simulink model "Line_Follower"  (R2024b)
settings: Solver=VariableStepAuto  StartTime=0.0  StopTime=360  RelTol=1e-3
settings Model: Creator=varun  LastModifiedBy=varun

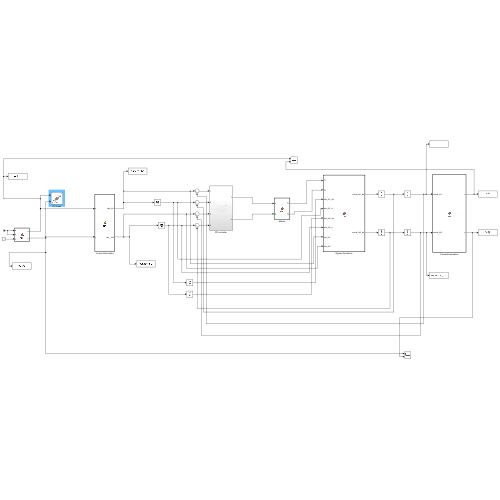
[thumbnail: Simulink's stored preview of the top-level diagram]
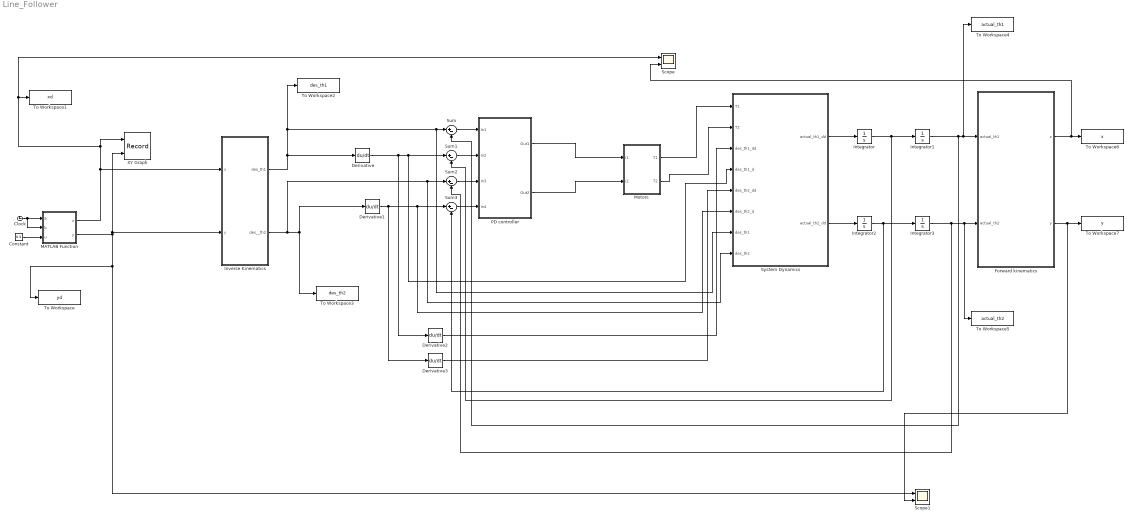
== system Line_Follower ==
  Clock : Clock
      settings: Decimation=360
  Constant : Constant  Value=0.3
  Derivative{,1..3} (4 alike) : Derivative
  Forward kinematics : MATLAB Function  TreatAsAtomicUnit=on
  Integrator{,1..3} (4 alike) : Integrator
  Inverse Kinematics : MATLAB Function  TreatAsAtomicUnit=on
  MATLAB Function : MATLAB Function  TreatAsAtomicUnit=on
  Motors : MATLAB Function  TreatAsAtomicUnit=on
  PD controller : Subsystem
  Scope : Scope  NumInputPorts=2
  Scope1 : Scope  NumInputPorts=2
  Sum{,1..3} (4 alike) : Sum  Inputs=|+-
  System Dynamics : MATLAB Function  TreatAsAtomicUnit=on
  To Workspace : ToWorkspace  VariableName=yd  SampleTime=-1
  To Workspace1 : ToWorkspace  VariableName=xd  SampleTime=-1
  To Workspace2 : ToWorkspace  VariableName=des_th1  SampleTime=-1
  To Workspace3 : ToWorkspace  VariableName=des_th2  SampleTime=-1
  To Workspace4 : ToWorkspace  VariableName=actual_th1  SampleTime=-1
  To Workspace5 : ToWorkspace  VariableName=actual_th2  SampleTime=-1
  To Workspace6 : ToWorkspace  VariableName=x  SampleTime=-1
  To Workspace7 : ToWorkspace  VariableName=y  SampleTime=-1
  XY Graph : Record  FileSettingsInternal="{\"entries\":[{\"content\":{\"excelSettings\":{\"content\":{},\"type\":\"Streamout.ExcelSettings\"}},\"type\":\"Streamout.FileSettingStorage\",\"uuid\":\"\"}],\"packageUris\":[\"http:\\/\\/schema.mathworks.com\\/mf0\\/streamout_blocks\\/R2020a\"],\"version\":\"1.0\"}"  Layout=[1 1]  SignalsInternal="{\"entries\":[{\"content\":{\"signals\":[{\"content\":{\"blockPath\":[],\"dimensions\":[1],\"domain\":\"\",\"lineColor\":\"#a2142f\",\"plots\":[ 1 ],\"port\":1,\"sid\":[\"\"],\"signalID\":1,\"signalName\":\"MATLAB Function:1\"},\"type\":\"RecordBlkView.Signal\",\"uuid\":\"\"},{\"content\":{\"blockPath\":[],\"dimensions\":[1],\"domain\":\"\",\"lineColor\":\"#139fff\",\"plots\":[ 1 ],\"port\":2,\"sid\":[\"\"],\"signalID\":2,\"signalName\":\"MATLAB Function:2\"},\"type\":\"RecordBlkView.Signal\",\"uuid\":\"\"}]},\"type\":\"RecordBlkView.InputSignals\",\"uuid\":\"\"}],\"packageUris\":[\"http:\\/\\/schema.mathworks.com\\/mf0\\/streamout_blocks\\/R2020a\"],\"version\":\"1.0\"}"  VisualizationBindings="{\"xyplotplugin\":{\"info\":[{\"series\":[{\"bindingParametersList\":[{\"parameter\":\"X-Axis\",\"signalID\":1,\"signalName\":\"MATLAB Function:1\"},{\"parameter\":\"Y-Axis\",\"signalID\":2,\"signalName\":\"MATLAB Function:2\"}],\"seriesID\":0}],\"subplotID\":1}]}}"  CompatibilityTag=XY
  wires:
  Constant/1 -> MATLAB Function/3(u)
  Clock/1 -> MATLAB Function/2(b), MATLAB Function/1(a)
  MATLAB Function/1(x) -> Inverse Kinematics/1(x), XY Graph/1, Scope/1, To Workspace1/1
  MATLAB Function/2(y) -> XY Graph/2, Inverse Kinematics/2(y), Scope1/1, To Workspace/1
  Inverse Kinematics/1(des_th1) -> To Workspace2/1, System Dynamics/7(des_th1), Sum/1, Derivative/1
  Derivative/1 -> System Dynamics/4(des_th1_d), Sum1/1, Derivative2/1
  Inverse Kinematics/2(des__th2) -> System Dynamics/8(des_th2), Sum2/1, To Workspace3/1, Derivative1/1
  Derivative1/1 -> Derivative3/1, System Dynamics/6(des_th2_d), Sum3/1
  Sum/1 -> PD controller/1(In1)
  Sum1/1 -> PD controller/2(In2)
  Sum2/1 -> PD controller/3(In3)
  Sum3/1 -> PD controller/4(In4)
  PD controller/1(Out1) -> Motors/1(i1)
  PD controller/2(Out2) -> Motors/2(i2)
  Motors/1(T1) -> System Dynamics/1(T1)
  Motors/2(T2) -> System Dynamics/2(T2)
  Derivative2/1 -> System Dynamics/3(des_th1_dd)
  Derivative3/1 -> System Dynamics/5(des_th2_dd)
  Integrator/1 -> Sum1/2, Integrator1/1
  Integrator2/1 -> Sum3/2, Integrator3/1
  System Dynamics/2(actual_th2_dd) -> Integrator2/1
  System Dynamics/1(actual_th1_dd) -> Integrator/1
  Integrator1/1 -> Sum/2, To Workspace4/1, Forward kinematics/1(actual_th1)
  Integrator3/1 -> Sum2/2, To Workspace5/1, Forward kinematics/2(actual_th2)
  Forward kinematics/2(y) -> Scope1/2, To Workspace7/1
  Forward kinematics/1(x) -> Scope/2, To Workspace6/1

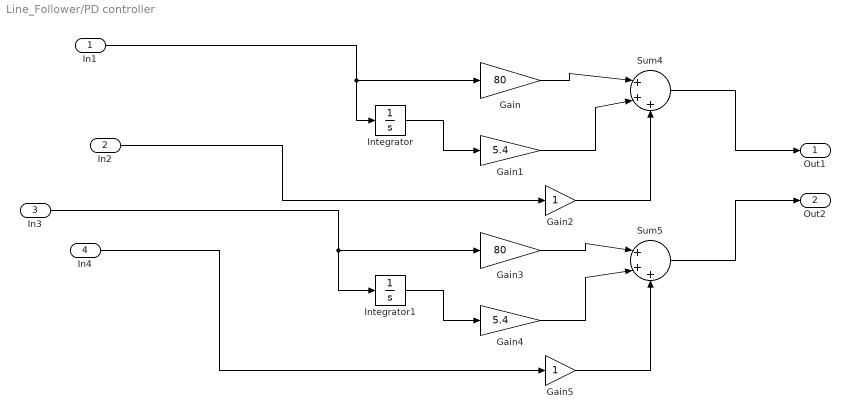
== system Line_Follower/PD controller ==
  In1 : Inport
  In2 : Inport  Port=2
  In3 : Inport  Port=3
  In4 : Inport  Port=4
  Gain : Gain  Gain=80
  Gain1 : Gain  Gain=5.4
  Gain2 : Gain
  Gain3 : Gain  Gain=80
  Gain4 : Gain  Gain=5.4
  Gain5 : Gain
  Integrator : Integrator
  Integrator1 : Integrator
  Sum4 : Sum  Inputs=|+++
  Sum5 : Sum  Inputs=|+++
  Out1 : Outport
  Out2 : Outport  Port=2
  wires:
  Gain4/1 -> Sum5/2
  Gain5/1 -> Sum5/3
  In3/1 -> Integrator1/1, Gain3/1
  Gain/1 -> Sum4/1
  Integrator1/1 -> Gain4/1
  Gain1/1 -> Sum4/2
  Gain3/1 -> Sum5/1
  Sum5/1 -> Out2/1
  Integrator/1 -> Gain1/1
  Sum4/1 -> Out1/1
  Gain2/1 -> Sum4/3
  In1/1 -> Integrator/1, Gain/1
  In2/1 -> Gain2/1
  In4/1 -> Gain5/1

== matlab function Line_Follower/Inverse Kinematics ==
  data: x input; y input; des_th1 output; des__th2 output
function [des_th1,des__th2]= fcn(x,y)
L1=2;
L2=1;
M1=1;
M2=0.5;
c2= (x^2 +y^2 -L1^2 -L2^2)/(2*L1*L2)
s2=(1-c2^2)^0.5
K1= L1+L2*c2
K2=L2*s2
des_th1= atan2 (y,x)-atan2(K2,K1);
des__th2=atan2 (s2,c2);

== matlab function Line_Follower/MATLAB Function ==
  data: a input; b input; x output; u input; y output
function [x, y] = fcn(a, b, u)

x = 1 + u*cosd(a);
y = 1 + u*sind(b);

== matlab function Line_Follower/Motors ==
  data: i1 input; T1 output; i2 input; T2 output
function [T1,T2]= fcn(i1,i2)
kt=10;
T1=kt*i1;
kt=10;
T2=kt*i2;

== matlab function Line_Follower/System Dynamics ==
  data: T1 input; actual_th1_dd output; T2 input; des_th1_dd input; des_th1_d input; des_th2_dd input; des_th2_d input; des_th1 input; des_th2 input; actual_th2_dd output
function [actual_th1_dd,actual_th2_dd]= fcn(T1, T2,des_th1_dd,des_th1_d,des_th2_dd,des_th2_d,des_th1,des_th2)



N=1;
jm1=0.01;
jm2=0.01;
cm1=0.1;
cm2=0.1;
M1=1;
M2=0.5;
L1=2;
L2=1;
g=9.8;

th1=des_th1
th2=des_th2
th1dd=des_th1_dd
th1d=des_th1_d
th2dd=des_th2_dd
th2d=des_th2_d

M=[((M1+M2)*(L1^2)+ (M2*L2^2)+ (2*M2*L1*L2*cos(th2)))  (M2*L2^2+ M2*L1*L2*cos(th2));
   (M2*L2^2+M2*L1*L2*cos(th2))                   (M2*L2^2)];


V=[((-M2*L1*L2)*(2*th1d*th2d+th2d^2)*sin(th2));
   (M2*L1*L2*th1d^2*sin(th2))];




 G= [((M1+M2)*g*L1*cos(th1)+M2*g*L2*cos(th1+th2));
     M2*g*L2*cos(th1+th2)];
 
 Tt1= N*T1 -N^2* jm1*des_th1_dd -N^2*cm1 *des_th1_d
 Tt2= N*T2 -N^2* jm2*des_th2_dd -N^2*cm2 *des_th2_d
 
NJ=[N*jm1 0;
   0 N*jm2]

NT=[N*T1;
N*T2]

NC=[N*cm1 0;
0 N*cm2]

thd=[des_th1_d;
des_th1_d]


actual_th_dd= inv(M+NJ) *(NT -V- G-(NC*thd));
v= actual_th_dd(1)
w=actual_th_dd(2)

actual_th1_dd=v
actual_th2_dd=w

== matlab function Line_Follower/Forward kinematics ==
  data: x output; actual_th1 input; y output; actual_th2 input
function [x,y]= fcn(actual_th1,actual_th2)

L1=2;
L2=1;


x=L2*cos(actual_th1 + actual_th2) + L1*cos(actual_th1)
y=L2*sin(actual_th1 + actual_th2) + L1*sin(actual_th1)
